simulink model "untitled"  (R2013b)
settings: Solver=ode45  StartTime=0.0  StopTime=10.0  RelTol=1e-3
values from neighbouring files (symbols this model uses):
  A = [-Bx 0 0 h1*sin(a1) h1*sin(a2) h1*sin(a3) h1*sin(a4) ... (first row only)    [SSLController.m]    (also in Untitled.m = [A;a]; aaa.m = zeros(7,7); avr.m = zeros(7,7); dynamicModel.m = zeros(11,11))
  B = [-sin(a1)*g1/m -sin(a2)*g1/m -sin(a3)*g1/m -sin(a4)*g1/m ... (first row only)    [SSLController.m]    (also in aaa.m = zeros(7,4); avr.m = zeros(7,4); dynamicModel.m = zeros(11,4); ssl_robot.m = zeros(7,4))
  C = eye(7)    [SSLController.m]    (also in aaa.m = eye(7,7); avr.m = eye(7,7); dynamicModel.m = eye(11,11); ssl_robot.m = eye(7,7))
  D = 0    [SSLController.m]    (also in aaa.m = zeros(7,4); avr.m = zeros(7,4); ssl_robot.m = zeros(7,4))
settings Model: Creator=QWA  LastModifiedBy=QWA

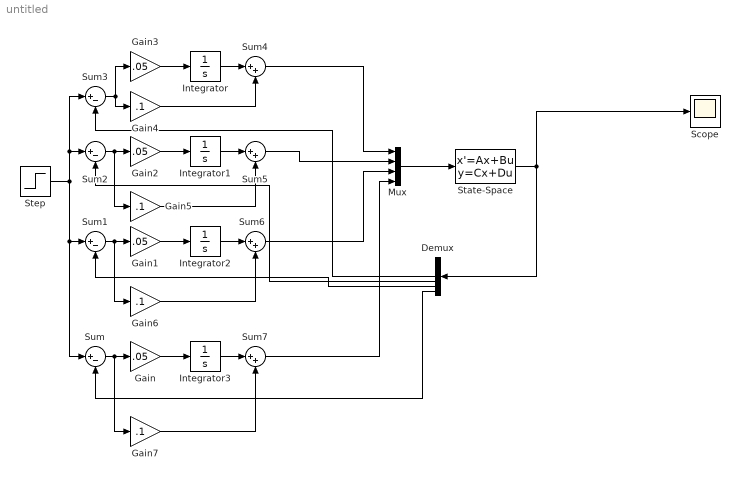
== system untitled ==
  Demux : Demux  Outputs=7
  Gain{,1..3} (4 alike) : Gain  Gain=.05
  Gain{4..7} (4 alike) : Gain  Gain=.1
  Integrator{,1..3} (4 alike) : Integrator
  Mux : Mux
  Scope : Scope
      settings: MaxDataPoints=50000  SampleInput=on
  State-Space : StateSpace  A=A  B=B  C=C  D=D  X0=0
  Step : Step  SampleTime=0
  Sum{,1..3} (4 alike) : Sum  Inputs=|+-
  Sum{4..7} (4 alike) : Sum  Inputs=|++
  wires:
  State-Space/1 -> Demux/1, Scope/1
  Mux/1 -> State-Space/1
  Demux/7 -> Sum/2
  Sum/1 -> Gain7/1, Gain/1
  Gain/1 -> Integrator3/1
  Demux/6 -> Sum1/2
  Sum1/1 -> Gain6/1, Gain1/1
  Gain1/1 -> Integrator2/1
  Demux/5 -> Sum2/2
  Sum2/1 -> Gain5/1, Gain2/1
  Gain2/1 -> Integrator1/1
  Step/1 -> Sum3/1, Sum2/1, Sum/1, Sum1/1
  Demux/4 -> Sum3/2
  Sum3/1 -> Gain4/1, Gain3/1
  Gain3/1 -> Integrator/1
  Integrator3/1 -> Sum7/1
  Gain4/1 -> Sum4/2
  Integrator/1 -> Sum4/1
  Sum4/1 -> Mux/1
  Integrator1/1 -> Sum5/1
  Sum5/1 -> Mux/2
  Gain5/1 -> Sum5/2
  Gain6/1 -> Sum6/2
  Integrator2/1 -> Sum6/1
  Sum6/1 -> Mux/3
  Gain7/1 -> Sum7/2
  Sum7/1 -> Mux/4
